simulink library "xbsReplacements_r4"  (Simulink 7.1)
undefined symbols (not defined in the file or in its folder): period, xlGetSimulinkPeriod
libraries: xbsIndex_r4 x223
(part 1 of 3)
settings Model: Creator=singhj  LastModifiedBy=sysgengroup

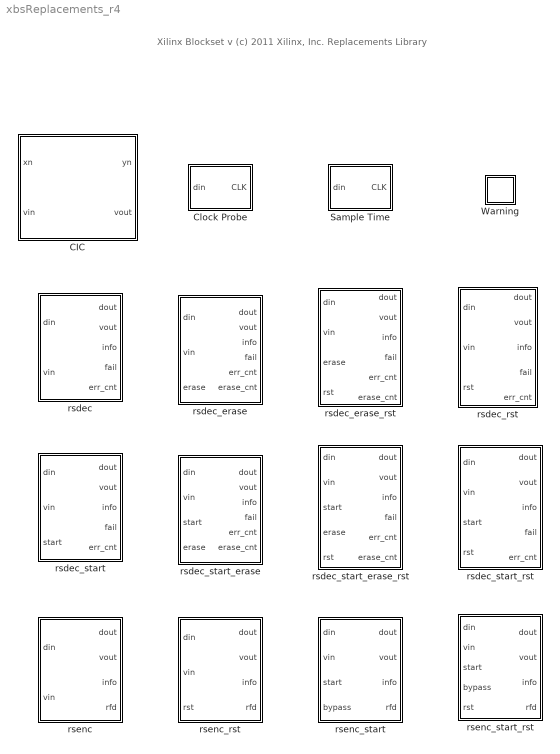
== system xbsReplacements_r4 ==
  note: Xilinx Blockset v
      | (c) 2011 Xilinx, Inc.
      |
      | Replacements Library
  CIC : Subsystem  mask{input_bitwidth=20, input_binpt=18, filter_type=Interpolator, samp_rate_change=8, stages=1, differential_delay=1, latency=1}
      mask prompts: input_bitwidth "Input Bit Width"; input_binpt "Input Binary Point"; filter_type "Filter Type"; samp_rate_change "Sample Rate Change"; stages "Number of Stages"; differential_delay "Differential Delay"
      mask init:
      | [bg,fg] = xlcmap('XBlock',0);
      | iPos = get_param(gcb,'Position');
      | iWidth=iPos(3)-iPos(1); iHeight=iPos(4)-iPos(2);
      | iCx=iWidth/2;
      | iCy=iHeight/2;
      | [logoX, logoY] = xlogo(iPos);
      | % Print label on the block
      | if(filter_type == 2)
      |    str = sprintf('%d-Stage\n CIC\n%d:1 Decimator',stages, samp_rate_change);
      | else
      |    str = sprintf('%d-Stage\n CIC\n1:%d Interpolator',stages, samp_rate_change);	
      | end
      | cic_blk = [gcb '/CIC Filter'];
      | 
      | switch filter_type
      |     case 1
      |         set_param(cic_blk, 'filter_type','Interpolator');
      |     otherwise
      |         set_param(cic_blk, 'filter_type','Decimator');
      | end
      | 
      | set_param(cic_blk, 'm',num2str(differential_delay));
      settings: CopyFcn=set_param(gcb, 'LinkStatus', 'none');
      mask StyleString: edit,edit,popup(Interpolator|Decimator),edit,edit,popup(1|2|3|4),edit
      mask Display:
      | patch([0 iWidth iWidth 0],[0 0 iHeight iHeight] , bg);
      | patch(logoX,logoY , fg);
      | plot([0 0 iWidth iWidth 0], [0 iHeight iHeight 0 0]);
      | disp(str);
      | 
      | port_label('input',1,'xn');
      | port_label('input',2,'vin');
      | 
      | port_label('output',1,'yn');
      | port_label('output',2,'vout');
  Clock Probe : Subsystem
      settings: CopyFcn=set_param(gcb, 'LinkStatus', 'none');
      mask Display: disp('CLK')
  Sample Time : Subsystem
      settings: CopyFcn=set_param(gcb, 'LinkStatus', 'none');
      mask Display: disp('ST')
  Warning : Subsystem  mask{period=period}
      settings: OpenFcn="warndlg(['This block used to set an explicit sample period of ''', get_param(gcb, 'period'), '''. With System Generator v8.1,  it is rare that rates need to be specified explicitly.', sprintf('\\n\\n'), 'If, after trying to simulate the updated diagram, you find that some rates do not resolve, you may need to insert one or more Assert blocks.', sprintf('\\n\\n'), 'NOTE: To quickly remove these triangular markers from your diagram, run: xlRmWarn(subsystem).'])"
      mask Display:
      | patch([0 1 .5 0], [.8 .8 0 .8], [.9 .95 .2]);
      | 
      | color('gray');
      | plot([0 1 .5 0], [.8 .8 0 .8]);
      | 
      | color('red');
      | disp('\fontsize{16pt}\bf!','texmode','on');
  rsdec : Subsystem
      settings: CopyFcn=set_param(gcb, 'LinkStatus', 'none');
  rsdec_erase : Subsystem
      settings: CopyFcn=set_param(gcb, 'LinkStatus', 'none');
  rsdec_erase_rst : Subsystem
      settings: CopyFcn=set_param(gcb, 'LinkStatus', 'none');
  rsdec_rst : Subsystem
      settings: CopyFcn=set_param(gcb, 'LinkStatus', 'none');
  rsdec_start : Subsystem
      settings: CopyFcn=set_param(gcb, 'LinkStatus', 'none');
  rsdec_start_erase : Subsystem
      settings: CopyFcn=set_param(gcb, 'LinkStatus', 'none');
  rsdec_start_erase_rst : Subsystem
      settings: CopyFcn=set_param(gcb, 'LinkStatus', 'none');
  rsdec_start_rst : Subsystem
      settings: CopyFcn=set_param(gcb, 'LinkStatus', 'none');
  rsenc : Subsystem
      settings: CopyFcn=set_param(gcb, 'LinkStatus', 'none');
  rsenc_rst : Subsystem
      settings: CopyFcn=set_param(gcb, 'LinkStatus', 'none');
  rsenc_start : Subsystem
      settings: CopyFcn=set_param(gcb, 'LinkStatus', 'none');
  rsenc_start_rst : Subsystem
      settings: CopyFcn=set_param(gcb, 'LinkStatus', 'none');

== system xbsReplacements_r4/CIC ==
  note: For the CIC filter to work in your design
      |  the "Input Bit Width" and "Input Binary Point"
      | for the CIC filter should be set on the mask
      | above this subsystem to match the input data
      | width and binary point.
  xn : Inport  OutDataType=sfix(16)  OutScaling=2^0
  vin : Inport  Port=2  OutDataType=sfix(16)  OutScaling=2^0
  Assert : xbsIndex_r4/Assert  assert_type=on  arith_type="Signed  (2's comp)"  n_bits=input_bitwidth  bin_pt=input_binpt  assert_rate=off  period=1  block_type=assert
      settings: infoedit=Asserts a user-defined sample rate and/or type on a signal.<P><P>Hardware notes: In hardware this block costs nothing.  block_version=VER_STRING_GOES_HERE
  CIC Filter : Subsystem  mask(CIC Filter){input_bitwidth=input_bitwidth, input_binpt=input_binpt, filter_type=Interpolator, rate_change=samp_rate_change, stages=stages, m=1, pipeline=on, dbl_ovrd=off}
      mask prompts: input_bitwidth "Input Bit Width"; input_binpt "Input Binary Point"; filter_type "Filter Type"; rate_change "Sample Rate Change"; stages "Number of Stages"; m "Differential Delay"; pipeline "Pipeline Differentiators"; dbl_ovrd "Override with Doubles"
      mask help: Cascaded Integrated Comb (CIC) Filter
      mask init:
      | % CIC Single Channel v1.0
      | % Set Block Logo
      | [bg,fg] = xlcmap('XBlock',dbl_ovrd);
      | iPos = get_param(gcb,'Position');
      | iWidth=iPos(3)-iPos(1); iHeight=iPos(4)-iPos(2);
      | iCx=iWidth/2;
      | iCy=iHeight/2;
      | [logoX, logoY] = xlogo(iPos);	
      | 
      | % Print label on the block
      | if(filter_type == 2)
      |    str = sprintf('%d-Stage\n CIC\n%d:1 Decimator',stages, rate_change);
      | else
      |    str = sprintf('%d-Stage\n CIC\n1:%d Interpolator',stages, rate_change);	
      | end
      | 
      | set_param(gcb, 'LinkStatus', 'none');
      | sav_gcb=gcb;
      | 
      | % Make sure the entered values for stages and channels are positive integers
      | nstages = round(sum(abs(stages)));
      | 
      | % Calculate previous filter type 0 = Decimator, 1 = Interpolator
      | pft = find_system(sav_gcb, 'lookUnderMasks', 'all', 'FollowLinks','on','Name', 'Up Sample');
      | prev_filter_type = length(pft(:,1));
      | 
      | %calculate how many stages currently in the model
      | a = find_system(sav_gcb, 'lookUnderMasks', 'all', 'FollowLinks','on','masktype', 'Integrator Stage');
      | d = find_system(sav_gcb, 'lookUnderMasks', 'all', 'FollowLinks','on','masktype', 'Differentiator Stage');
      | prev_stages = length(a(:,1));
      | 
      | % issue an error if the number of stages entered is zero
      | if (nstages == 0)
      | 	nstages = prev_stages;
      | 	errordlg('Number of Stages must be more that zero')
      | end
      | 
      | if(filter_type == 2) % Decimator
      |    
      | 	
      |    if (prev_filter_type == 1) % was interpolator so turn to decimator
      | 	
      | 	  % disconnect all the wires from all the blocks
      |        for i= 2:prev_stages,
      | 	      delete_line(sav_gcb, ['Integrator' int2str(i-1) '/' int2str(1)], ['Integrator' int2str(i) '/' int2str(1)]);
      | 	      delete_line(sav_gcb, ['Differentiator' int2str(i-1) '/' int2str(1)], ['Differentiator' int2str(i) '/' int2str(1)]);
      |        end
      | 
      |        % disconnect the last blocks in the two sections
      |        delete_line(sav_gcb, ['Differentiator' int2str(prev_stages) '/' int2str(1)], ['Up Sample/1']);
      |        delete_line(sav_gcb, ['Integrator' int2str(prev_stages) '/' int2str(1)], 'Out1/1');
      | 	
      | 	   % delete the line from the Up sampler to the Integrator
      | 	   delete_line(sav_gcb, 'Up Sample/1', 'Integrator1/1'); 
      | 	   delete_line(sav_gcb, 'In1/1', 'Differentiator1/1'); 
      | 	   
      | 	   % Delete the Up Sampler and then replace with an Down Sampler
      | 	   pup = get_param([sav_gcb '/Up Sample'], 'position');
      | 	   delete_block([sav_gcb '/Up Sample']);
      | 	   load_system('xbsIndex_r4');
      | 	   add_block('xbsIndex_r4/Down Sample', [sav_gcb '/Down Sample'], 'sample_ratio', 'rate_change','sample_phase', 'First Value of Frame', 'position', [pup(1), pup(2), pup(3),pup(4)]);
      | 	   
      | 	   % Switch the Integrators and Decimators around
      | 	   for i=1:prev_stages,
      | 		   tempi = get_param([sav_gcb '/Integrator' int2str(i)], 'position');
      | 	       tempd = get_param([sav_gcb '/Differentiator' int2str(i)], 'position');
      | 		   set_param([sav_gcb '/Differentiator' int2str(i)], 'position', [tempi(1), tempi(2), tempi(3), tempi(4)], 'output_bitwidth', 'ceil(stages*log2(rate_change*m) + input_bitwidth)');
      | 		   set_param([sav_gcb '/Integrator' int2str(i)], 'position', [tempd(1), tempd(2), tempd(3), tempd(4)]);
      | 	   end
      | 	   	   	
      | 	   % add back in the lines
      |        add_line(sav_gcb, 'In1/1', 'Integrator1/1', 'autorouting', 'on');
      | 	   add_line(sav_gcb, ['Integrator' int2str(prev_stages) '/1'], 'Down Sample/1', 'autorouting', 'on');
      | 	   add_line(sav_gcb, 'Down Sample/1', 'Differentiator1/1', 'autorouting', 'on');
      | 	   add_line(sav_gcb, ['Differentiator' int2str(prev_stages) '/1'], 'Out1/1', 'autorouting', 'on');
      | 	   for i= 2:prev_stages,
      |           add_line(sav_gcb, ['Integrator' int2str(i-1) '/1'], ['Integrator' int2str(i) '/' int2str(1)], 'autorouting', 'on');
      |           add_line(sav_gcb, ['Differentiator' int2str(i-1) '/1'], ['Differentiator' int2str(i) '/' int2str(1)], 'autorouting', 'on');
      | 	   end
      | 		
      |        %Set the Output bit widths of Differentiator and Integrator stages
      |        set_param([sav_gcb '/Differentiator1'], 'output_bitwidth', 'ceil(stages*log2(rate_change*m) + input_bitwidth)');
      | 	   	   %Set the Output bit width of Integrator stages
      | 	   %Calculate the Interpolator Integrator Output Bit Growth
      |        for i= 1:nstages,
      | 			 j = nstages+i;
      | 	         set_param([sav_gcb '/Integrator' int2str(i)], 'output_bitwidth', 'ceil(stages*log2(rate_change*m) + input_bitwidth)');
      |              set_param([sav_gcb '/Differentiator' int2str(i)], 'output_bitwidth', 'ceil(stages*log2(rate_change*m) + input_bitwidth)');
      | 	   end
      | 	   
      |    end
      |    
      |    if (nstages ~= prev_stages)
      |     
      |        % disconnect all the wires from all the blocks
      |        for i= 2:prev_stages,
      | 	      delete_line(sav_gcb, ['Integrator' int2str(i-1) '/' int2str(1)], ['Integrator' int2str(i) '/' int2str(1)]);
      | 	      delete_line(sav_gcb, ['Differentiator' int2str(i-1) '/' int2str(1)], ['Differentiator' int2str(i) '/' int2str(1)]);
      |        end
      | 
      |        % disconnect the last blocks in the two sections
      |        delete_line(sav_gcb, ['Integrator' int2str(prev_stages) '/' int2str(1)], ['Down Sample/1']);
      |        delete_line(sav_gcb, ['Differentiator' int2str(prev_stages) '/' int2str(1)], 'Out1/1');
      | 	
      | 	   % delete the line from the down sampler to the differentiator
      | 	   delete_line(sav_gcb, 'Down Sample/1', 'Differentiator1/1');
      | 	
      | 	   % Remove all the blocks except the first one (as we always will have one)
      |        for i=2:prev_stages,
      | 		  delete_block([sav_gcb '/Differentiator' int2str(i)]);
      | 	      delete_block([sav_gcb '/Integrator' int2str(i)]);
      |        end
      | 	   
      | 	   %Set the Output bit width of Differentiator stages
      |        set_param([sav_gcb '/Differentiator1'], 'output_bitwidth', 'ceil(stages*log2(rate_change*m) + input_bitwidth)');
      | 	   
      | 	   % collect data on the position of existing blocks
      | 	   pi = get_param([sav_gcb '/Integrator1'], 'position');
      | 	   pd = get_param([sav_gcb '/Differentiator1'], 'position');
      | 	   set_param([sav_gcb '/Differentiator1'], 'position', [pi(1)+(nstages+1)*80, pd(2), pi(3)+(nstages+1)*80, pd(4)]);
      | 	   pd = get_param([sav_gcb '/Differentiator1'], 'position');
      | 	
      | 	   % move the current blocks to accomadate for new blocks to be added 
      | 	   pds = get_param([sav_gcb '/Down Sample'], 'position');
      | 	   set_param([sav_gcb '/Down Sample'], 'position', [pi(1)+(nstages)*80, pds(2), pi(3)+(nstages)*80, pds(4)]);
      | 	   
      | 	   po = get_param([sav_gcb '/Out1'], 'position');
      | 	   set_param([sav_gcb '/Out1'], 'position', [pd(1)+(nstages+1)*80, po(2), pd(1)+(po(3)-po(1))+(nstages+1)*80, po(4)]);	
      | 	
      | 	   % add back in the line between the Down Sampler and the 1st Differentiator
      |        add_line(sav_gcb, 'Down Sample/1', ['Differentiator1/' int2str(1)], 'autorouting', 'on');
      | 
      | 	   % Only add blocks if more than one stage is required
      | 	   if (nstages ~= 1)
      | 		
      | 	       % Add in a copy of the first block to make up the required number of stages
      |            for i=2:nstages,
      |                add_block([sav_gcb '/Integrator1'], [sav_gcb '/Integrator' int2str(i)], 'position', [pi(1)+(i-1)*80, pi(2), pi(3)+(i-1)*80, pi(4)]);
      | 		       add_block([sav_gcb '/Differentiator1'], [sav_gcb '/Differentiator' int2str(i)], 'position', [pd(1)+(i-1)*80, pd(2), pd(3)+(i-1)*80, pd(4)]);
      | 	       end
      | 		
      | 	       % Connect up the wires to each block use autorouting
      |            for i= 2:nstages,
      |  		       add_line(sav_gcb, ['Integrator' int2str(i-1) '/' int2str(1)], ['Integrator' int2str(i) '/' int2str(1)], 'autorouting', 'on');
      | 	           add_line(sav_gcb, ['Differentiator' int2str(i-1) '/' int2str(1)], ['Differentiator' int2str(i) '/' int2str(1)], 'autorouting', 'on');
      |            end
      | 	    end
      | 	       % Connect the last blocks in the two sections
      |            add_line(sav_gcb, ['Integrator' int2str(nstages) '/' int2str(1)], ['Down Sample/1'], 'autorouting', 'on');
      |            add_line(sav_gcb, ['Differentiator' int2str(nstages) '/' int2str(1)], ['Out1/1'], 'autorouting', 'on');
      |    end
      | 
      | else % Interpolator
      |    
      | 	
      | 	if (prev_filter_type == 0) % was decimator so turn to interpolator
      | 	
      | 	  % disconnect all the wires from all the blocks
      |        for i= 2:prev_stages,
      | 	      delete_line(sav_gcb, ['Integrator' int2str(i-1) '/' int2str(1)], ['Integrator' int2str(i) '/' int2str(1)]);
      | 	      delete_line(sav_gcb, ['Differentiator' int2str(i-1) '/' int2str(1)], ['Differentiator' int2str(i) '/' int2str(1)]);
      |        end
      | 
      |        % disconnect the last blocks in the two sections
      |        delete_line(sav_gcb, ['Integrator' int2str(prev_stages) '/' int2str(1)], ['Down Sample/1']);
      |        delete_line(sav_gcb, ['Differentiator' int2str(prev_stages) '/' int2str(1)], 'Out1/1');
      | 	
      | 	   % delete the line from the down sampler to the Differentiator
      | 	   delete_line(sav_gcb, 'Down Sample/1', 'Differentiator1/1'); 
      | 	   delete_line(sav_gcb, 'In1/1', 'Integrator1/1'); 
      | 	   
      | 	   % Delete the Down Sampler and then replace with a Up Sampler
      | 	   pdwn = get_param([sav_gcb '/Down Sample'], 'position');
      | 	   delete_block([sav_gcb '/Down Sample']);
      | 	   load_system('xbsIndex_r4');
      | 	   add_block('xbsIndex_r4/Up Sample', [sav_gcb '/Up Sample'], 'sample_ratio', 'rate_change', 'position', [pdwn(1), pdwn(2), pdwn(3), pdwn(4)]);
      | 	   
      | 	   % Switch the Integrators and Decimators around
      | 	   for i=1:prev_stages,
      | 		   tempi = get_param([sav_gcb '/Integrator' int2str(i)], 'position');
      | 	       tempd = get_param([sav_gcb '/Differentiator' int2str(i)], 'position');
      | 		   set_param([sav_gcb '/Differentiator' int2str(i)], 'position', [tempi(1), tempi(2), tempi(3), tempi(4)], 'output_bitwidth', [int2str(i) '+ input_bitwidth']);
      | 		   set_param([sav_gcb '/Integrator' int2str(i)], 'position', [tempd(1), tempd(2), tempd(3), tempd(4)]);
      | 	   end
      | 	   	   	
      | 	   % add back in the lines
      |        add_line(sav_gcb, 'In1/1', 'Differentiator1/1', 'autorouting', 'on');
      | 	   add_line(sav_gcb, ['Differentiator' int2str(prev_stages) '/1'], 'Up Sample/1', 'autorouting', 'on');
      | 	   add_line(sav_gcb, 'Up Sample/1', 'Integrator1/1', 'autorouting', 'on');
      | 	   add_line(sav_gcb, ['Integrator' int2str(prev_stages) '/1'], 'Out1/1', 'autorouting', 'on');
      | 	   for i= 2:prev_stages,
      |           add_line(sav_gcb, ['Integrator' int2str(i-1) '/1'], ['Integrator' int2str(i) '/1'], 'autorouting', 'on');
      |           add_line(sav_gcb, ['Differentiator' int2str(i-1) '/1'], ['Differentiator' int2str(i) '/1'], 'autorouting', 'on');
      | 	   end
      | 	   
      | 	   %Set the Output bit width of Integrator stages
      | 	   %Calculate the Interpolator Integrator Output Bit Growth
      |        for i= 1:nstages,
      | 			 j = nstages+i;
      | 	         set_param([sav_gcb '/Integrator' int2str(i)], 'output_bitwidth', ['ceil(log2(2^(2*stages-' int2str(j) ')*(rate_change*m)^(' int2str(j) '-stages)) + input_bitwidth)']);
      | 	   end
      | 		
      |    end
      |    
      | 	
      | 	if (nstages ~= prev_stages)
      |     
      |        % disconnect all the wires from all the blocks
      |        for i= 2:prev_stages,
      | 	      delete_line(sav_gcb, ['Integrator' int2str(i-1) '/' int2str(1)], ['Integrator' int2str(i) '/' int2str(1)]);
      | 	      delete_line(sav_gcb, ['Differentiator' int2str(i-1) '/' int2str(1)], ['Differentiator' int2str(i) '/' int2str(1)]);
      |        end
      | 
      |        % disconnect the last blocks in the two sections
      |        delete_line(sav_gcb, ['Differentiator' int2str(prev_stages) '/' int2str(1)], ['Up Sample/1']);
      |        delete_line(sav_gcb, ['Integrator' int2str(prev_stages) '/' int2str(1)], 'Out1/1');
      |        
      | 	
      | 	   % delete the line from the Up sampler to the Integrator1 for movement later
      | 	   delete_line(sav_gcb, 'Up Sample/1', 'Integrator1/1'); 
      | 	
      | 	   % Remove all the blocks except the first one (as we always will have one)
      |        for i=2:prev_stages,
      | 		  delete_block([sav_gcb '/Differentiator' int2str(i)]);
      | 	      delete_block([sav_gcb '/Integrator' int2str(i)]);
      |        end
      | 	
      | 	   %Set the Output bit width of first Differentiator stage (other are set as copies of this block)
      |        set_param([sav_gcb '/Differentiator1'], 'output_bitwidth', '1 + input_bitwidth');
      | 	   
      | 	   % collect data on the position of existing blocks
      | 	   pi = get_param([sav_gcb '/Integrator1'], 'position');
      | 	   pd = get_param([sav_gcb '/Differentiator1'], 'position');
      | 	   set_param([sav_gcb '/Integrator1'], 'position', [pd(1)+(nstages+1)*80, pi(2), pd(3)+(nstages+1)*80, pi(4)]);
      | 	   pi = get_param([sav_gcb '/Integrator1'], 'position');
      | 	
      | 	   % move the current blocks to accomadate for new blocks to be added 
      | 	   pus = get_param([sav_gcb '/Up Sample'], 'position');
      | 	   set_param([sav_gcb '/Up Sample'], 'position', [pd(1)+(nstages)*80, pus(2), pd(3)+(nstages)*80, pus(4)]);
      | 	
      | 	   po = get_param([sav_gcb '/Out1'], 'position');
      |        set_param([sav_gcb '/Out1'], 'position', [pi(1)+(nstages+1)*80, po(2), pi(1)+(po(3)-po(1))+(nstages+1)*80, po(4)]);	
      |       
      | 	
      | 	   % add back in the line between the Up Sampler and the 1st Integrator1
      | 	   add_line(sav_gcb, 'Up Sample/1', 'Integrator1/1', 'autorouting', 'on');
      | 	   
      | 	   % Only add blocks if more than one stage is required
      | 	   if (nstages ~= 1)
      | 		
      | 	       % Add in a copy of the first block to make up the required number of stages
      |            for i=2:nstages,
      |                add_block([sav_gcb '/Integrator1'], [sav_gcb '/Integrator' int2str(i)], 'position', [pi(1)+(i-1)*80, pi(2), pi(3)+(i-1)*80, pi(4)]);
      | 		       add_block([sav_gcb '/Differentiator1'], [sav_gcb '/Differentiator' int2str(i)], 'position', [pd(1)+(i-1)*80, pd(2), pd(3)+(i-1)*80, pd(4)], 'output_bitwidth', [int2str(i) '+ input_bitwidth']);
      | 	       end
      | 		
      | 	       % Connect up the wires to each block use autorouting
      |            for i= 2:nstages,
      |  		       add_line(sav_gcb, ['Integrator' int2str(i-1) '/' int2str(1)], ['Integrator' int2str(i) '/' int2str(1)], 'autorouting', 'on');
      | 	           add_line(sav_gcb, ['Differentiator' int2str(i-1) '/' int2str(1)], ['Differentiator' int2str(i) '/' int2str(1)], 'autorouting', 'on');
      |            end
      | 	    end
      | 	       % Connect the last blocks in the two sections
      |            add_line(sav_gcb, ['Differentiator' int2str(nstages) '/1'], ['Up Sample/1'], 'autorouting', 'on');
      |            add_line(sav_gcb, ['Integrator' int2str(nstages) '/1'], ['Out1/1'], 'autorouting', 'on');
      | 		   
      | 	     %Set the Output bit width of Integrator stages
      | 	     %Calculate the Interpolator Integrator Output Bit Growth
      |           for i= 1:nstages,
      | 			 j = nstages+i;
      | 	         set_param([sav_gcb '/Integrator' int2str(i)], 'output_bitwidth', ['ceil(log2(2^(2*stages-' int2str(j) ')*(rate_change*m)^(' int2str(j) '-stages)) + input_bitwidth)']);
      | 	      end
      |    end
      | 	  
      | end
      | 
      | 
      | % Set the pipelining to ON or OFF on the differentiators
      | if (pipeline == 0)
      | 	for i= 1:nstages
      | 		set_param([sav_gcb '/Differentiator' int2str(i), '/AddSub'], 'latency', '0')
      | 	end
      | else
      | 	for i= 1:nstages
      | 		set_param([sav_gcb '/Differentiator' int2str(i), '/AddSub'], 'latency' ,'1')
      | 	end
      | end
      | 
      | % Set the overide with doubles on with selected
      | % Find all the Xilinx Blocks in the system
      | total = find_system(sav_gcb, 'lookUnderMasks', 'all', 'FollowLinks','on','Blocktype', 'S-Function');
      | total_length = length(total(:,1));
      | 
      | if (dbl_ovrd == 0)
      | 	for i= 1:total_length,
      |     	set_param(char(total(i)), 'dbl_ovrd', 'off');
      | 	end
      | else
      | 	for i= 1:total_length,
      | 		set_param(char(total(i)), 'dbl_ovrd', 'on');
      | 	end
      | 	[bg,fg]=xlcmap('XBlock',1);
      | end
      settings: CopyFcn=set_param(gcb, 'LinkStatus', 'none');
      mask Help: eval('xlWeb(xlhtmldoclink(''CIC Filter''))');
      mask StyleString: edit,edit,popup(Interpolator|Decimator),edit,edit,popup(1|2|3|4),checkbox,checkbox
      mask Display:
      | patch([0 iWidth iWidth 0],[0 0 iHeight iHeight] , bg);
      | patch(logoX,logoY , fg);
      | plot([0 0 iWidth iWidth 0], [0 iHeight iHeight 0 0]);
      | disp(str)
  Delay : xbsIndex_r4/Delay  en=off  latency=latency-1  dbl_ovrd=off  reg_retiming=off  block_type=delay
      settings: infoedit=Hardware notes: A delay line is a chain, each link of which is an SRL16 followed by a flip-flop. If register retiming is enabled, the delay line is a chain of flip-flops.  block_version=VER_STRING_GOES_HERE
  Delay1 : xbsIndex_r4/Delay  en=off  latency=latency  dbl_ovrd=off  reg_retiming=off  block_type=delay
      settings: infoedit=Hardware notes: A delay line is a chain, each link of which is an SRL16 followed by a flip-flop. If register retiming is enabled, the delay line is a chain of flip-flops.  block_version=VER_STRING_GOES_HERE
  Subsystem2 : Subsystem
  Terminator : Terminator
  yn : Outport  OutDataType=sfix(16)  OutScaling=2^0
  vout : Outport  Port=2  OutDataType=sfix(16)  OutScaling=2^0
  wires:
  Delay1/1 -> vout/1
  Delay/1 -> yn/1
  CIC Filter/1(Out1) -> Delay/1, Subsystem2/1(sample)
  xn/1 -> Assert/1
  vin/1 -> Terminator/1
  Subsystem2/1(const) -> Delay1/1
  Assert/1 -> CIC Filter/1(In1)

== system xbsReplacements_r4/Clock Probe ==
  din : Inport  OutDataType=sfix(16)  OutScaling=2^0
  Clock Probe : xbsIndex_r4/Clock Probe  block_type=clkprobe
      settings: infoedit="Clock probe.  Produces an output of type double that mirrors the hardware system clock.<P><P>Hardware notes:  This block is ignored when hardware is generated."  block_version=VER_STRING_GOES_HERE
  Terminator : Terminator
  CLK : Outport  OutDataType=sfix(16)  OutScaling=2^0
  wires:
  din/1 -> Terminator/1
  Clock Probe/1 -> CLK/1

== system xbsReplacements_r4/Sample Time ==
  din : Inport  OutDataType=sfix(16)  OutScaling=2^0
  Gain : Gain  Gain=xlGetSimulinkPeriod(gcb)  ParameterDataType=sfix(16)  ParameterScaling=2^0  OutDataType=sfix(16)  OutScaling=2^0
  Sample Time : xbsIndex_r4/Sample Time  block_type=sampletime
      settings: infoedit=The Sample Time block reports the sample period of its input.<P><P>Hardware notes: This block is implemented as a constant in hardware.  block_version=VER_STRING_GOES_HERE
  CLK : Outport  OutDataType=sfix(16)  OutScaling=2^0
  wires:
  din/1 -> Sample Time/1
  Sample Time/1 -> Gain/1
  Gain/1 -> CLK/1

== system xbsReplacements_r4/Warning ==

== system xbsReplacements_r4/rsdec ==
  note: Note: In earlier versions of System Generator, RS Decoder was programmed to always support
      |           continuous code processing. This was done by oversampling the RS decoder and setting
      |           the Clocks Per Symbol to be a value greater than 1. In this version of System Generator, this value
      |           has to be set explicitly for supporting continuous code decoding. Refer to the RS Decoder
      |           implementation in sysgenConcatenatedFEC demo to see a example of how to set the RS decoder to
      |           have clocks per symbol greater than 1. In this example, the RS decoder has specified clocks
      |           per symbol value of 8. The RS decoder is set to run at the system rate by upsampling the inputs by 8
      |          and downsampling the output by 8 'to match the data path rate.
  din : Inport  OutDataType=sfix(16)  OutScaling=2^0
  vin : Inport  Port=2  OutDataType=sfix(16)  OutScaling=2^0
  RS Decoder : xbsIndex_r4/RS Decoder v5_1   code_spec=Custom  num_channels=1  clocks_per_symbol=1  erase=off  data_del=off  n_in=off  rst=off  en=off  sym_width=8  nn=204  kk=188  poly_char=[ 1 0 0 0 1 1 1 0 1]  gen_start=0  scale=1  mem_style=Automatic  opt_mode=Speed  self_recovering=off  use_rpm=off  block_type=rsdecode
      settings: infoedit=Decodes systematically encoded RS codes. The decoder supports marking received data symbols as erasures.  block_version=VER_STRING_GOES_HERE
  Register : xbsIndex_r4/Register  init=1  rst=off  en=off  dbl_ovrd=off  block_type=register
      settings: block_version=VER_STRING_GOES_HERE
  Subsystem3 : Subsystem
  Terminator : Terminator
  Terminator1 : Terminator
  Terminator2 : Terminator
  info_generator : Subsystem  mask{sym_width=8, kk=188}
      mask prompts: sym_width "Symbol Width"; kk "Number of information symbols per code block"
  dout : Outport  OutDataType=sfix(16)  OutScaling=2^0
  vout : Outport  Port=2  OutDataType=sfix(16)  OutScaling=2^0
  info : Outport  Port=3  OutDataType=sfix(16)  OutScaling=2^0
  fail : Outport  Port=4  OutDataType=sfix(16)  OutScaling=2^0
  err_cnt : Outport  Port=5  OutDataType=sfix(16)  OutScaling=2^0
  wires:
  Subsystem3/1(const) -> Register/1
  Register/1 -> RS Decoder/3, info_generator/3(reset)
  din/1 -> RS Decoder/1, Subsystem3/1(sample)
  vin/1 -> RS Decoder/2
  RS Decoder/1 -> dout/1
  RS Decoder/6 -> fail/1
  RS Decoder/4 -> Terminator/1
  RS Decoder/8 -> Terminator1/1
  RS Decoder/5 -> err_cnt/1
  RS Decoder/3 -> info_generator/2(blk_end)
  RS Decoder/2 -> info_generator/1(blk_strt)
  info_generator/1(vout) -> vout/1
  info_generator/2(info) -> info/1
  RS Decoder/7 -> Terminator2/1

== system xbsReplacements_r4/rsdec_erase ==
  note: Note: In earlier versions of System Generator, RS Decoder was programmed to always support
      |           continuous code processing. This was done by oversampling the RS decoder and setting
      |           the Clocks Per Symbol to be a value greater than 1. In this version of System Generator, this value
      |           has to be set explicitly for supporting continuous code decoding. Refer to the RS Decoder
      |           implementation in sysgenConcatenatedFEC demo to see a example of how to set the RS decoder to
      |           have clocks per symbol greater than 1. In this example, the RS decoder has specified clocks
      |           per symbol value of 8. The RS decoder is set to run at the system rate by upsampling the inputs by 8
      |          and downsampling the output by 8 'to match the data path rate.
  din : Inport  OutDataType=sfix(16)  OutScaling=2^0
  vin : Inport  Port=2  OutDataType=sfix(16)  OutScaling=2^0
  erase : Inport  Port=3  OutDataType=sfix(16)  OutScaling=2^0
  RS Decoder : xbsIndex_r4/RS Decoder v5_1   code_spec=Custom  num_channels=1  clocks_per_symbol=1  erase=on  data_del=off  n_in=off  rst=off  en=off  sym_width=8  nn=204  kk=188  poly_char=[ 1 0 0 0 1 1 1 0 1]  gen_start=0  scale=1  mem_style=Automatic  opt_mode=Speed  self_recovering=off  use_rpm=off  block_type=rsdecode
      settings: infoedit=Decodes systematically encoded RS codes. The decoder supports marking received data symbols as erasures.  block_version=VER_STRING_GOES_HERE
  Register : xbsIndex_r4/Register  init=1  rst=off  en=off  dbl_ovrd=off  block_type=register
      settings: block_version=VER_STRING_GOES_HERE
  Subsystem3 : Subsystem
  Terminator : Terminator
  Terminator1 : Terminator
  Terminator2 : Terminator
  info_generator : Subsystem  mask{sym_width=8, kk=188}
      mask prompts: sym_width "Symbol Width"; kk "Number of information symbols per code block"
      settings: CopyFcn=set_param(gcb, 'LinkStatus', 'none');
  dout : Outport  OutDataType=sfix(16)  OutScaling=2^0
  vout : Outport  Port=2  OutDataType=sfix(16)  OutScaling=2^0
  info : Outport  Port=3  OutDataType=sfix(16)  OutScaling=2^0
  fail : Outport  Port=4  OutDataType=sfix(16)  OutScaling=2^0
  err_cnt : Outport  Port=5  OutDataType=sfix(16)  OutScaling=2^0
  erase_cnt : Outport  Port=6  OutDataType=sfix(16)  OutScaling=2^0
  wires:
  info_generator/2(info) -> info/1
  RS Decoder/2 -> info_generator/1(blk_strt)
  RS Decoder/3 -> info_generator/2(blk_end)
  RS Decoder/5 -> err_cnt/1
  RS Decoder/8 -> Terminator1/1
  RS Decoder/4 -> Terminator/1
  RS Decoder/6 -> fail/1
  RS Decoder/1 -> dout/1
  vin/1 -> RS Decoder/2
  din/1 -> RS Decoder/1, Subsystem3/1(sample)
  Register/1 -> RS Decoder/3, info_generator/3(reset)
  Subsystem3/1(const) -> Register/1
  erase/1 -> RS Decoder/4
  RS Decoder/9 -> erase_cnt/1
  RS Decoder/7 -> Terminator2/1
  info_generator/1(vout) -> vout/1

== system xbsReplacements_r4/rsdec_erase_rst ==
  note: Note: In earlier versions of System Generator, RS Decoder was programmed to always support
      |           continuous code processing. This was done by oversampling the RS decoder and setting
      |           the Clocks Per Symbol to be a value greater than 1. In this version of System Generator, this value
      |           has to be set explicitly for supporting continuous code decoding. Refer to the RS Decoder
      |           implementation in sysgenConcatenatedFEC demo to see a example of how to set the RS decoder to
      |           have clocks per symbol greater than 1. In this example, the RS decoder has specified clocks
      |           per symbol value of 8. The RS decoder is set to run at the system rate by upsampling the inputs by 8
      |          and downsampling the output by 8 'to match the data path rate.
  din : Inport  OutDataType=sfix(16)  OutScaling=2^0
  vin : Inport  Port=2  OutDataType=sfix(16)  OutScaling=2^0
  erase : Inport  Port=3  OutDataType=sfix(16)  OutScaling=2^0
  rst : Inport  Port=4  OutDataType=sfix(16)  OutScaling=2^0
  RS Decoder : xbsIndex_r4/RS Decoder v5_1   code_spec=Custom  num_channels=1  clocks_per_symbol=1  erase=on  data_del=off  n_in=off  rst=on  en=off  sym_width=8  nn=204  kk=188  poly_char=[ 1 0 0 0 1 1 1 0 1]  gen_start=0  scale=1  mem_style=Automatic  opt_mode=Speed  self_recovering=off  use_rpm=off  block_type=rsdecode
      settings: infoedit=Decodes systematically encoded RS codes. The decoder supports marking received data symbols as erasures.  block_version=VER_STRING_GOES_HERE
  Register : xbsIndex_r4/Register  init=1  rst=off  en=off  dbl_ovrd=off  block_type=register
      settings: block_version=VER_STRING_GOES_HERE
  Subsystem3 : Subsystem
  Terminator : Terminator
  Terminator1 : Terminator
  Terminator2 : Terminator
  info_generator : Subsystem  mask{sym_width=8, kk=188}
      mask prompts: sym_width "Symbol Width"; kk "Number of information symbols per code block"
  dout : Outport  OutDataType=sfix(16)  OutScaling=2^0
  vout : Outport  Port=2  OutDataType=sfix(16)  OutScaling=2^0
  info : Outport  Port=3  OutDataType=sfix(16)  OutScaling=2^0
  fail : Outport  Port=4  OutDataType=sfix(16)  OutScaling=2^0
  err_cnt : Outport  Port=5  OutDataType=sfix(16)  OutScaling=2^0
  erase_cnt : Outport  Port=6  OutDataType=sfix(16)  OutScaling=2^0
  wires:
  info_generator/1(vout) -> vout/1
  RS Decoder/7 -> Terminator2/1
  RS Decoder/9 -> erase_cnt/1
  erase/1 -> RS Decoder/4
  Subsystem3/1(const) -> Register/1
  Register/1 -> RS Decoder/3, info_generator/3(reset)
  din/1 -> RS Decoder/1, Subsystem3/1(sample)
  vin/1 -> RS Decoder/2
  RS Decoder/1 -> dout/1
  RS Decoder/6 -> fail/1
  RS Decoder/4 -> Terminator/1
  RS Decoder/8 -> Terminator1/1
  RS Decoder/5 -> err_cnt/1
  RS Decoder/3 -> info_generator/2(blk_end)
  RS Decoder/2 -> info_generator/1(blk_strt)
  info_generator/2(info) -> info/1
  rst/1 -> RS Decoder/5, info_generator/4(rst)

== system xbsReplacements_r4/rsdec_rst ==
  note: Note: In earlier versions of System Generator, RS Decoder was programmed to always support
      |           continuous code processing. This was done by oversampling the RS decoder and setting
      |           the Clocks Per Symbol to be a value greater than 1. In this version of System Generator, this value
      |           has to be set explicitly for supporting continuous code decoding. Refer to the RS Decoder
      |           implementation in sysgenConcatenatedFEC demo to see a example of how to set the RS decoder to
      |           have clocks per symbol greater than 1. In this example, the RS decoder has specified clocks
      |           per symbol value of 8. The RS decoder is set to run at the system rate by upsampling the inputs by 8
      |          and downsampling the output by 8 'to match the data path rate.
  din : Inport  OutDataType=sfix(16)  OutScaling=2^0
  vin : Inport  Port=2  OutDataType=sfix(16)  OutScaling=2^0
  rst : Inport  Port=3  OutDataType=sfix(16)  OutScaling=2^0
  RS Decoder : xbsIndex_r4/RS Decoder v5_1   code_spec=Custom  num_channels=1  clocks_per_symbol=1  erase=off  data_del=off  n_in=off  rst=on  en=off  sym_width=8  nn=204  kk=188  poly_char=[1 1 0 0 0 0 1 1 1]  gen_start=112  scale=11  mem_style=Automatic  opt_mode=Speed  self_recovering=off  use_rpm=on  block_type=rsdecode
      settings: infoedit=Decodes systematically encoded RS codes. The decoder supports marking received data symbols as erasures.  xl_area=[0, 0, 0, 0, 0, 0, 0]  block_version=VER_STRING_GOES_HERE
  Register : xbsIndex_r4/Register  init=1  rst=off  en=off  dbl_ovrd=off  block_type=register
      settings: block_version=VER_STRING_GOES_HERE
  Subsystem3 : Subsystem
  Terminator : Terminator
  Terminator1 : Terminator
  Terminator2 : Terminator
  info_generator : Subsystem  mask{sym_width=8, kk=188}
      mask prompts: sym_width "Symbol Width"; kk "Number of information symbols per code block"
  dout : Outport  OutDataType=sfix(16)  OutScaling=2^0
  vout : Outport  Port=2  OutDataType=sfix(16)  OutScaling=2^0
  info : Outport  Port=3  OutDataType=sfix(16)  OutScaling=2^0
  fail : Outport  Port=4  OutDataType=sfix(16)  OutScaling=2^0
  err_cnt : Outport  Port=5  OutDataType=sfix(16)  OutScaling=2^0
  wires:
  rst/1 -> info_generator/4(rst), RS Decoder/4
  Subsystem3/1(const) -> Register/1
  Register/1 -> RS Decoder/3, info_generator/3(reset)
  din/1 -> RS Decoder/1, Subsystem3/1(sample)
  vin/1 -> RS Decoder/2
  RS Decoder/1 -> dout/1
  RS Decoder/6 -> fail/1
  RS Decoder/4 -> Terminator/1
  RS Decoder/8 -> Terminator1/1
  RS Decoder/5 -> err_cnt/1
  RS Decoder/3 -> info_generator/2(blk_end)
  RS Decoder/2 -> info_generator/1(blk_strt)
  RS Decoder/7 -> Terminator2/1
  info_generator/2(info) -> info/1
  info_generator/1(vout) -> vout/1

== system xbsReplacements_r4/rsdec_start ==
  note: Note: In earlier versions of System Generator, RS Decoder was programmed to always support
      |           continuous code processing. This was done by oversampling the RS decoder and setting
      |           the Clocks Per Symbol to be a value greater than 1. In this version of System Generator, this value
      |           has to be set explicitly for supporting continuous code decoding. Refer to the RS Decoder
      |           implementation in sysgenConcatenatedFEC demo to see a example of how to set the RS decoder to
      |           have clocks per symbol greater than 1. In this example, the RS decoder has specified clocks
      |           per symbol value of 8. The RS decoder is set to run at the system rate by upsampling the inputs by 8
      |          and downsampling the output by 8 'to match the data path rate.
  din : Inport  OutDataType=sfix(16)  OutScaling=2^0
  vin : Inport  Port=2  OutDataType=sfix(16)  OutScaling=2^0
  start : Inport  Port=3  OutDataType=sfix(16)  OutScaling=2^0
  RS Decoder : xbsIndex_r4/RS Decoder v5_1   code_spec=Custom  num_channels=1  clocks_per_symbol=1  erase=off  data_del=off  n_in=off  rst=off  en=off  sym_width=8  nn=204  kk=188  poly_char=[ 1 0 0 0 1 1 1 0 1]  gen_start=0  scale=1  mem_style=Automatic  opt_mode=Speed  self_recovering=off  use_rpm=off  block_type=rsdecode
      settings: infoedit=Decodes systematically encoded RS codes. The decoder supports marking received data symbols as erasures.  block_version=VER_STRING_GOES_HERE
  Register : xbsIndex_r4/Register  init=1  rst=off  en=off  dbl_ovrd=off  block_type=register
      settings: block_version=VER_STRING_GOES_HERE
  Subsystem3 : Subsystem
  Terminator : Terminator
  Terminator1 : Terminator
  Terminator2 : Terminator
  expr : xbsIndex_r4/Expression  expression=a & b  align_bp=on  en=off  latency=0  precision=Full  arith_type=Unsigned  n_bits=8  bin_pt=2  dbl_ovrd=off  block_type=expr
      settings: block_version=VER_STRING_GOES_HERE
  info_generator : Subsystem  mask{sym_width=8, kk=188}
      mask prompts: sym_width "Symbol Width"; kk "Number of information symbols per code block"
      settings: CopyFcn=set_param(gcb, 'LinkStatus', 'none');
  dout : Outport  OutDataType=sfix(16)  OutScaling=2^0
  vout : Outport  Port=2  OutDataType=sfix(16)  OutScaling=2^0
  info : Outport  Port=3  OutDataType=sfix(16)  OutScaling=2^0
  fail : Outport  Port=4  OutDataType=sfix(16)  OutScaling=2^0
  err_cnt : Outport  Port=5  OutDataType=sfix(16)  OutScaling=2^0
  wires:
  RS Decoder/2 -> info_generator/1(blk_strt)
  RS Decoder/3 -> info_generator/2(blk_end)
  RS Decoder/5 -> err_cnt/1
  RS Decoder/8 -> Terminator1/1
  RS Decoder/4 -> Terminator/1
  RS Decoder/6 -> fail/1
  RS Decoder/7 -> Terminator2/1
  RS Decoder/1 -> dout/1
  din/1 -> RS Decoder/1, Subsystem3/1(sample)
  Register/1 -> RS Decoder/3, info_generator/3(reset)
  Subsystem3/1(const) -> Register/1
  expr/1 -> RS Decoder/2
  vin/1 -> expr/1
  start/1 -> expr/2
  info_generator/2(info) -> info/1
  info_generator/1(vout) -> vout/1

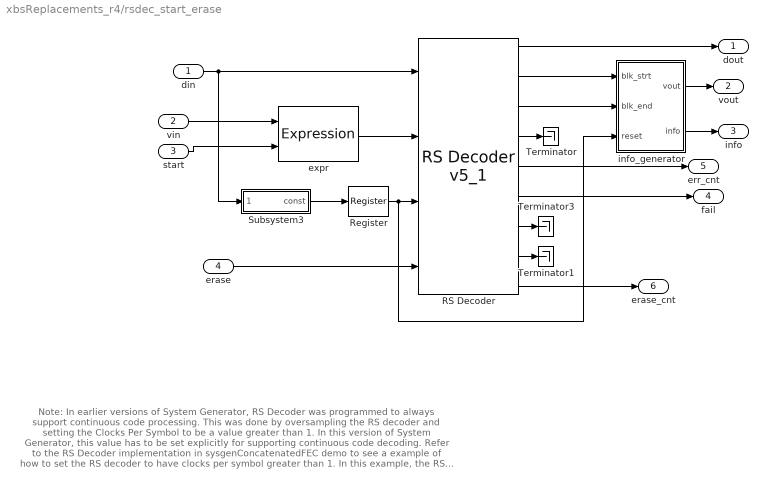
== system xbsReplacements_r4/rsdec_start_erase ==
  note: Note: In earlier versions of System Generator, RS Decoder was programmed to always support
      |           continuous code processing. This was done by oversampling the RS decoder and setting
      |           the Clocks Per Symbol to be a value greater than 1. In this version of System Generator, this value
      |           has to be set explicitly for supporting continuous code decoding. Refer to the RS Decoder
      |           implementation in sysgenConcatenatedFEC demo to see a example of how to set the RS decoder to
      |           have clocks per symbol greater than 1. In this example, the RS decoder has specified clocks
      |           per symbol value of 8. The RS decoder is set to run at the system rate by upsampling the inputs by 8
      |          and downsampling the output by 8 'to match the data path rate.
  din : Inport  OutDataType=sfix(16)  OutScaling=2^0
  vin : Inport  Port=2  OutDataType=sfix(16)  OutScaling=2^0
  start : Inport  Port=3  OutDataType=sfix(16)  OutScaling=2^0
  erase : Inport  Port=4  OutDataType=sfix(16)  OutScaling=2^0
  RS Decoder : xbsIndex_r4/RS Decoder v5_1   code_spec=Custom  num_channels=1  clocks_per_symbol=1  erase=on  data_del=off  n_in=off  rst=off  en=off  sym_width=8  nn=204  kk=188  poly_char=[ 1 0 0 0 1 1 1 0 1]  gen_start=0  scale=1  mem_style=Automatic  opt_mode=Speed  self_recovering=off  use_rpm=off  block_type=rsdecode
      settings: infoedit=Decodes systematically encoded RS codes. The decoder supports marking received data symbols as erasures.  block_version=VER_STRING_GOES_HERE
  Register : xbsIndex_r4/Register  init=1  rst=off  en=off  dbl_ovrd=off  block_type=register
      settings: block_version=VER_STRING_GOES_HERE
  Subsystem3 : Subsystem
  Terminator : Terminator
  Terminator1 : Terminator
  Terminator3 : Terminator
  expr : xbsIndex_r4/Expression  expression=a & b  align_bp=on  en=off  latency=0  precision=Full  arith_type=Unsigned  n_bits=8  bin_pt=2  dbl_ovrd=off  block_type=expr
      settings: block_version=VER_STRING_GOES_HERE
  info_generator : Subsystem  mask{sym_width=8, kk=188}
      mask prompts: sym_width "Symbol Width"; kk "Number of information symbols per code block"
      settings: CopyFcn=set_param(gcb, 'LinkStatus', 'none');
  dout : Outport  OutDataType=sfix(16)  OutScaling=2^0
  vout : Outport  Port=2  OutDataType=sfix(16)  OutScaling=2^0
  info : Outport  Port=3  OutDataType=sfix(16)  OutScaling=2^0
  fail : Outport  Port=4  OutDataType=sfix(16)  OutScaling=2^0
  err_cnt : Outport  Port=5  OutDataType=sfix(16)  OutScaling=2^0
  erase_cnt : Outport  Port=6  OutDataType=sfix(16)  OutScaling=2^0
  wires:
  start/1 -> expr/2
  vin/1 -> expr/1
  expr/1 -> RS Decoder/2
  Subsystem3/1(const) -> Register/1
  Register/1 -> RS Decoder/3, info_generator/3(reset)
  din/1 -> RS Decoder/1, Subsystem3/1(sample)
  RS Decoder/1 -> dout/1
  RS Decoder/6 -> fail/1
  RS Decoder/4 -> Terminator/1
  RS Decoder/8 -> Terminator1/1
  RS Decoder/5 -> err_cnt/1
  RS Decoder/3 -> info_generator/2(blk_end)
  RS Decoder/2 -> info_generator/1(blk_strt)
  erase/1 -> RS Decoder/4
  RS Decoder/9 -> erase_cnt/1
  RS Decoder/7 -> Terminator3/1
  info_generator/2(info) -> info/1
  info_generator/1(vout) -> vout/1

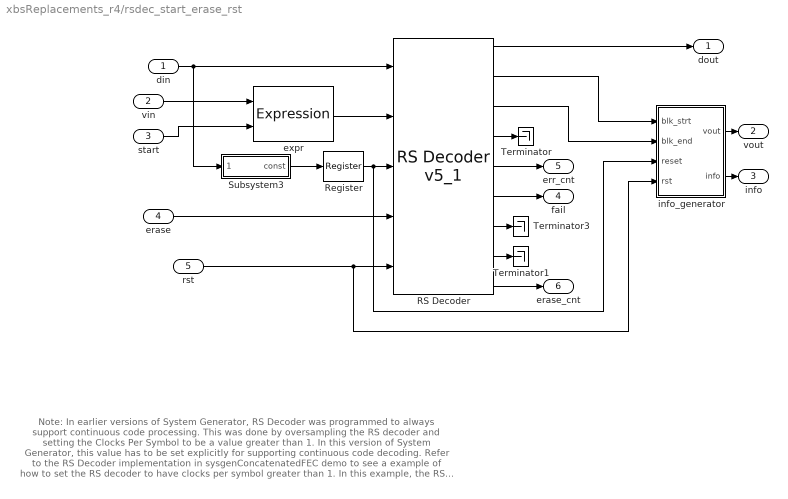
== system xbsReplacements_r4/rsdec_start_erase_rst ==
  note: Note: In earlier versions of System Generator, RS Decoder was programmed to always support
      |           continuous code processing. This was done by oversampling the RS decoder and setting
      |           the Clocks Per Symbol to be a value greater than 1. In this version of System Generator, this value
      |           has to be set explicitly for supporting continuous code decoding. Refer to the RS Decoder
      |           implementation in sysgenConcatenatedFEC demo to see a example of how to set the RS decoder to
      |           have clocks per symbol greater than 1. In this example, the RS decoder has specified clocks
      |           per symbol value of 8. The RS decoder is set to run at the system rate by upsampling the inputs by 8
      |          and downsampling the output by 8 'to match the data path rate.
  din : Inport  OutDataType=sfix(16)  OutScaling=2^0
  vin : Inport  Port=2  OutDataType=sfix(16)  OutScaling=2^0
  start : Inport  Port=3  OutDataType=sfix(16)  OutScaling=2^0
  erase : Inport  Port=4  OutDataType=sfix(16)  OutScaling=2^0
  rst : Inport  Port=5  OutDataType=sfix(16)  OutScaling=2^0
  RS Decoder : xbsIndex_r4/RS Decoder v5_1   code_spec=Custom  num_channels=1  clocks_per_symbol=1  erase=on  data_del=off  n_in=off  rst=on  en=off  sym_width=8  nn=204  kk=188  poly_char=[ 1 0 0 0 1 1 1 0 1]  gen_start=0  scale=1  mem_style=Automatic  opt_mode=Speed  self_recovering=off  use_rpm=off  block_type=rsdecode
      settings: infoedit=Decodes systematically encoded RS codes. The decoder supports marking received data symbols as erasures.  block_version=VER_STRING_GOES_HERE
  Register : xbsIndex_r4/Register  init=1  rst=off  en=off  dbl_ovrd=off  block_type=register
      settings: block_version=VER_STRING_GOES_HERE
  Subsystem3 : Subsystem
  Terminator : Terminator
  Terminator1 : Terminator
  Terminator3 : Terminator
  expr : xbsIndex_r4/Expression  expression=a & b  align_bp=on  en=off  latency=0  precision=Full  arith_type=Unsigned  n_bits=8  bin_pt=2  dbl_ovrd=off  block_type=expr
      settings: block_version=VER_STRING_GOES_HERE
  info_generator : Subsystem  mask{sym_width=8, kk=188}
      mask prompts: sym_width "Symbol Width"; kk "Number of information symbols per code block"
  dout : Outport  OutDataType=sfix(16)  OutScaling=2^0
  vout : Outport  Port=2  OutDataType=sfix(16)  OutScaling=2^0
  info : Outport  Port=3  OutDataType=sfix(16)  OutScaling=2^0
  fail : Outport  Port=4  OutDataType=sfix(16)  OutScaling=2^0
  err_cnt : Outport  Port=5  OutDataType=sfix(16)  OutScaling=2^0
  erase_cnt : Outport  Port=6  OutDataType=sfix(16)  OutScaling=2^0
  wires:
  RS Decoder/9 -> erase_cnt/1
  erase/1 -> RS Decoder/4
  RS Decoder/2 -> info_generator/1(blk_strt)
  RS Decoder/3 -> info_generator/2(blk_end)
  RS Decoder/5 -> err_cnt/1
  RS Decoder/8 -> Terminator1/1
  RS Decoder/4 -> Terminator/1
  RS Decoder/6 -> fail/1
  RS Decoder/1 -> dout/1
  din/1 -> RS Decoder/1, Subsystem3/1(sample)
  Register/1 -> RS Decoder/3, info_generator/3(reset)
  Subsystem3/1(const) -> Register/1
  expr/1 -> RS Decoder/2
  vin/1 -> expr/1
  start/1 -> expr/2
  rst/1 -> info_generator/4(rst), RS Decoder/5
  info_generator/1(vout) -> vout/1
  info_generator/2(info) -> info/1
  RS Decoder/7 -> Terminator3/1

== system xbsReplacements_r4/rsdec_start_rst ==
  note: Note: In earlier versions of System Generator, RS Decoder was programmed to always support
      |           continuous code processing. This was done by oversampling the RS decoder and setting
      |           the Clocks Per Symbol to be a value greater than 1. In this version of System Generator, this value
      |           has to be set explicitly for supporting continuous code decoding. Refer to the RS Decoder
      |           implementation in sysgenConcatenatedFEC demo to see a example of how to set the RS decoder to
      |           have clocks per symbol greater than 1. In this example, the RS decoder has specified clocks
      |           per symbol value of 8. The RS decoder is set to run at the system rate by upsampling the inputs by 8
      |          and downsampling the output by 8 'to match the data path rate.
  din : Inport  OutDataType=sfix(16)  OutScaling=2^0
  vin : Inport  Port=2  OutDataType=sfix(16)  OutScaling=2^0
  start : Inport  Port=3  OutDataType=sfix(16)  OutScaling=2^0
  rst : Inport  Port=4  OutDataType=sfix(16)  OutScaling=2^0
  RS Decoder : xbsIndex_r4/RS Decoder v5_1   code_spec=Custom  num_channels=1  clocks_per_symbol=1  erase=off  data_del=off  n_in=off  rst=on  en=off  sym_width=8  nn=204  kk=188  poly_char=[ 1 0 0 0 1 1 1 0 1]  gen_start=0  scale=1  mem_style=Automatic  opt_mode=Speed  self_recovering=off  use_rpm=off  block_type=rsdecode
      settings: infoedit=Decodes systematically encoded RS codes. The decoder supports marking received data symbols as erasures.  block_version=VER_STRING_GOES_HERE
  Register : xbsIndex_r4/Register  init=1  rst=off  en=off  dbl_ovrd=off  block_type=register
      settings: block_version=VER_STRING_GOES_HERE
  Subsystem3 : Subsystem
  Terminator : Terminator
  Terminator1 : Terminator
  Terminator2 : Terminator
  expr : xbsIndex_r4/Expression  expression=a & b  align_bp=on  en=off  latency=0  precision=Full  arith_type=Unsigned  n_bits=8  bin_pt=2  dbl_ovrd=off  block_type=expr
      settings: block_version=VER_STRING_GOES_HERE
  info_generator : Subsystem  mask{sym_width=8, kk=188}
      mask prompts: sym_width "Symbol Width"; kk "Number of information symbols per code block"
  dout : Outport  OutDataType=sfix(16)  OutScaling=2^0
  vout : Outport  Port=2  OutDataType=sfix(16)  OutScaling=2^0
  info : Outport  Port=3  OutDataType=sfix(16)  OutScaling=2^0
  fail : Outport  Port=4  OutDataType=sfix(16)  OutScaling=2^0
  err_cnt : Outport  Port=5  OutDataType=sfix(16)  OutScaling=2^0
  wires:
  info_generator/1(vout) -> vout/1
  info_generator/2(info) -> info/1
  start/1 -> expr/2
  vin/1 -> expr/1
  expr/1 -> RS Decoder/2
  Subsystem3/1(const) -> Register/1
  Register/1 -> RS Decoder/3, info_generator/3(reset)
  din/1 -> RS Decoder/1, Subsystem3/1(sample)
  RS Decoder/1 -> dout/1
  RS Decoder/7 -> Terminator2/1
  RS Decoder/6 -> fail/1
  RS Decoder/4 -> Terminator/1
  RS Decoder/8 -> Terminator1/1
  RS Decoder/5 -> err_cnt/1
  RS Decoder/3 -> info_generator/2(blk_end)
  RS Decoder/2 -> info_generator/1(blk_strt)
  rst/1 -> info_generator/4(rst), RS Decoder/4
